simulink model "test_lianerized_model"  (R2026a)
settings: Solver=VariableStepAuto
undefined symbols (not defined in the file or in its folder): Sim
settings Model: Creator=Kiril  LastModifiedBy=Kiril

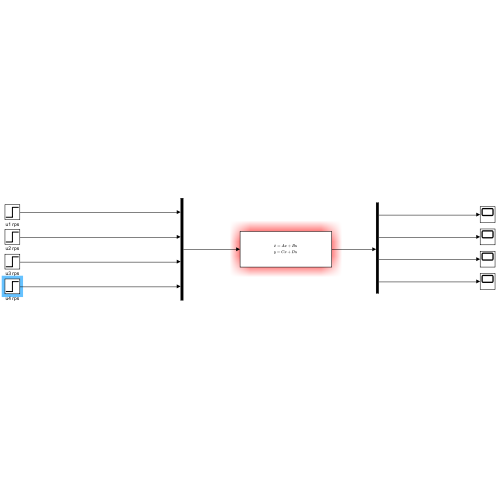
[thumbnail: Simulink's stored preview of the top-level diagram]
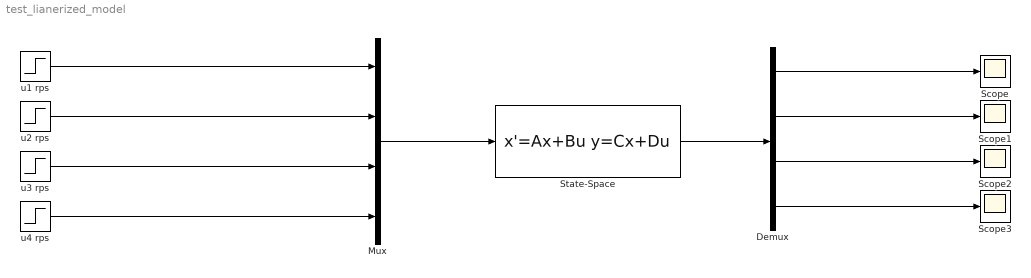
== system test_lianerized_model ==
  Demux : Demux
  Mux : Mux
  Scope{,1..3} (4 alike) : Scope
      Scope settings: ActiveDisplayYMinimum=-10.788055741836288  ActiveDisplayYMaximum=102.69648961273138
      Scope1 settings: ActiveDisplayYMinimum=-10.911370328691724  ActiveDisplayYMaximum=6.68963211623635
      Scope2 settings: ActiveDisplayYMinimum=-1.3989221715709474  ActiveDisplayYMaximum=1.1305947384443227  DataLoggingVariableName=ScopeData2
      Scope3 settings: ActiveDisplayYMinimum=-0.71445453253243962  ActiveDisplayYMaximum=3.2940558587020412  DataLoggingVariableName=ScopeData3
  State-Space : StateSpace  A=Sim.A  B=Sim.B  C=Sim.C  D=Sim.D  InitialCondition=Sim.initial_conditions
  u1 rps : Step  SampleTime=0
  u2 rps : Step  SampleTime=0
  u3 rps : Step  SampleTime=0
  u4 rps : Step  SampleTime=0
  wires:
  State-Space/1 -> Demux/1
  Demux/1 -> Scope/1
  Demux/2 -> Scope1/1
  Demux/3 -> Scope2/1
  Demux/4 -> Scope3/1
  Mux/1 -> State-Space/1
  u1 rps/1 -> Mux/1
  u2 rps/1 -> Mux/2
  u3 rps/1 -> Mux/3
  u4 rps/1 -> Mux/4
